simulink model "FlashMemory"  (R2016b)
settings: Solver=FixedStepAuto  StartTime=0.0  StopTime=10.0  RelTol=1e-3
PreLoadFcn:
  | waijung.modelPreload; % Required for working with Waijung Blockset. Do not remove.
undefined symbols (not defined in the file): CPHA_1Edge, CPOL_Low, deg_, Duplex, FirstBit_MSB, Full, g, imu, Link, LQFP100, ST, STM32F407VG, STM32F4DISCOVERY, Ts
libraries: simulink x45, stm32f4_i2c_lib x12, stm32f4_spi_lib x4, stm32f4_flash_lib x3, stm32f4_io_lib x1, cube_lib x1, stm32f4_device_config_lib x1, BC_USB x1
(part 3 of 3)

== matlab function FlashMemory/Read IMU/Bias Estimation IMU3 ==
  data: gyro input single; gyro_out output
function gyro_out = bias_estimation(gyro)

% For know we only use gyro around x, thus bias estimation for know is only
% on that measurment

persistent w_IMU3;
persistent w_bias_IMU3;
persistent bias_samples_IMU3;

n_samples = 250;

% init
if isempty(w_IMU3)
    w_IMU3 = zeros(3,n_samples,'single');
    w_bias_IMU3 = zeros(3,1,'single');
    bias_samples_IMU3 = 1;
end

% Take measurment for one second
if bias_samples_IMU3 < n_samples
    w_IMU3(:,bias_samples_IMU3) = gyro;       % Save all measurment in a vector
    bias_samples_IMU3 = bias_samples_IMU3 + 1;    % Increase counter
    gyro_out = zeros(3,1,'single');                 % Set output equal to zero

% After n_samples of measurement
elseif bias_samples_IMU3 == n_samples        
    w_bias_IMU3  = mean(w_IMU3,2,'native');                % Calculate the mean of the measurment
    bias_samples_IMU3 = bias_samples_IMU3 + 1;    % Increase counter
    gyro_out = gyro - w_bias_IMU3;                % Set output equal to zero
    
% When bias is cauclauted
else
    gyro_out = gyro - w_bias_IMU3;    % Subtract the bias from measurment
end

== matlab function FlashMemory/Read IMU/Bias Estimation IMU1 ==
  data: gyro input single; gyro_out output
function gyro_out = bias_estimation(gyro)

% For know we only use gyro around x, thus bias estimation for know is only
% on that measurment

persistent w_IMU1;
persistent w_bias_IMU1;
persistent bias_samples_IMU1;

n_samples = 250;

% init
if isempty(w_IMU1)
    w_IMU1 = zeros(3,n_samples,'single');
    w_bias_IMU1 = zeros(3,1,'single');
    bias_samples_IMU1 = 1;
end

% Take measurment for one second
if bias_samples_IMU1 < n_samples
    w_IMU1(:,bias_samples_IMU1) = gyro;       % Save all measurment in a vector
    bias_samples_IMU1 = bias_samples_IMU1 + 1;    % Increase counter
    gyro_out = zeros(3,1,'single');                 % Set output equal to zero

% After n_samples of measurement
elseif bias_samples_IMU1 == n_samples        
    w_bias_IMU1  = mean(w_IMU1,2,'native');                % Calculate the mean of the measurment
    bias_samples_IMU1 = bias_samples_IMU1 + 1;    % Increase counter
    gyro_out = gyro - w_bias_IMU1;                % Set output equal to zero
    
% When bias is cauclauted
else
    gyro_out = gyro - w_bias_IMU1;    % Subtract the bias from measurment
end

== matlab function FlashMemory/Read IMU/Accelometer Gyroscope I2C1/Read Accelometer and Gyroscope Data/Old gyro get data Used during SPI before/Take away Sensor fail reading ==
  data: y output; new input; old input
function y = fcn(new, old)
%#codegen
if(new > -257 && new < -200)
   y = old;
else
    y = new;
end

== matlab function FlashMemory/Read IMU/Accelometer Gyroscope I2C1/Read Accelometer and Gyroscope Data/Old gyro get data Used during SPI before/Take away Sensor fail reading if two bad in raw ==
  data: y output; new input; old input
function y = fcn(new, old)
%#codegen
if(new > -257 && new < -200)
   y = old;
else
    y = new;
end

== matlab function FlashMemory/Read IMU/Accelometer Gyroscope I2C1/Read Accelometer and Gyroscope Data/Old gyro get data Used during SPI before/Take away Sensor fail reading if two bad in raw1 ==
  data: y output; new input; old input
function y = fcn(new, old)
%#codegen
if(new > -257 && new < -200)
   y = old;
else
    y = new;
end

== matlab function FlashMemory/Read IMU/Accelometer Gyroscope I2C1/Read Accelometer and Gyroscope Data/Old gyro get data Used during SPI before/Take away Sensor fail reading1 ==
  data: y output; new input; old input
function y = fcn(new, old)
%#codegen
if(new > -257 && new < -200)
   y = old;
else
    y = new;
end

== matlab function FlashMemory/Read IMU/Accelometer Gyroscope I2C1/Read Accelometer and Gyroscope Data/Old gyro get data Used during SPI before/Take away Sensor fail reading if two bad in raw2 ==
  data: y output; new input; old input
function y = fcn(new, old)
%#codegen
if(new > -257 && new < -200)
   y = old;
else
    y = new;
end

== matlab function FlashMemory/Read IMU/Accelometer Gyroscope I2C1/Read Accelometer and Gyroscope Data/Old gyro get data Used during SPI before/Take away Sensor fail reading2 ==
  data: y output; new input; old input
function y = fcn(new, old)
%#codegen
if(new > -257 && new < -200)
   y = old;
else
    y = new;
end
